simulink model "q1_adaptive_controller_simulink"  (R2019a)
settings: Solver=VariableStepAuto  StartTime=0.0  StopTime=20  RelTol=1e-3
values from neighbouring files (symbols this model uses):
  alfa_1 = L*m*g    (= 9.8)    [q1_adaptive_controller_workspce.m]
  alfa_2 = k*L^2    (= 1)    [q1_adaptive_controller_workspce.m]
  alfa_3 = c*L^2    (= 1)    [q1_adaptive_controller_workspce.m]
  gama = 5    [q1_adaptive_controller_workspce.m]
  J = 2*L^2/3*m    (= 0.666666666667)    [q1_adaptive_controller_workspce.m]
  K = 10    [q1_adaptive_controller_workspce.m]
  lamda_0 = 5    [q1_adaptive_controller_workspce.m]
  Ts = 0.001    [q1_adaptive_controller_workspce.m]
libraries: simulink x1
settings Model: Creator=ronil  LastModifiedBy=ronil

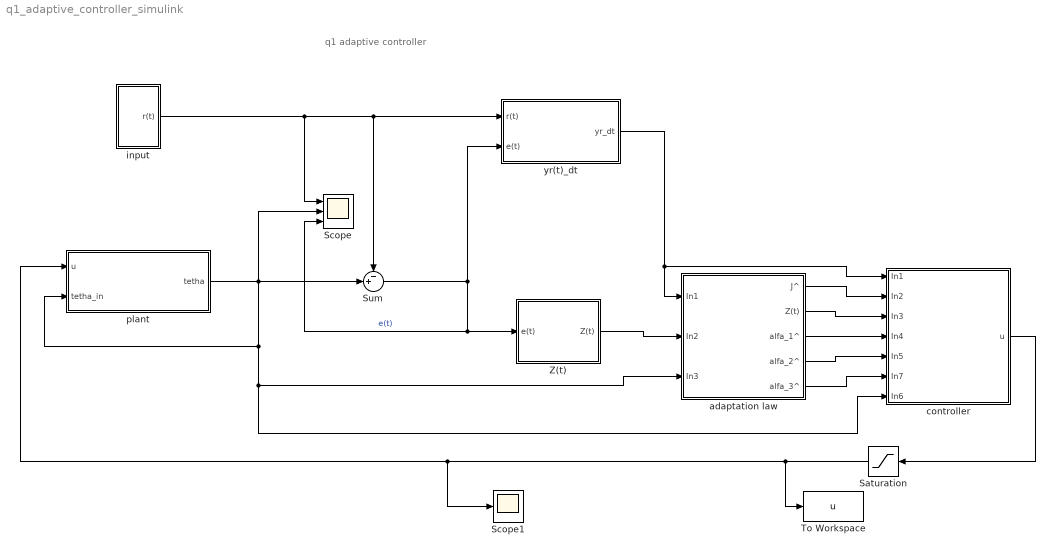
== system q1_adaptive_controller_simulink ==
  note: q1 adaptive controller
  Saturation : Saturate  UpperLimit=100000  LowerLimit=-100000  LinearizeAsGain=off  ZeroCross=off
  Scope : Scope  NumInputPorts=3
  Scope1 : Scope
  Sum : Sum  Inputs=-+|
  To Workspace : ToWorkspace  VariableName=u  SaveFormat=Timeseries  SampleTime=Ts
  Z(t) : Subsystem
  adaptation law : Subsystem
  controller : Subsystem
  input : Subsystem
  plant : Subsystem
  yr(t)_dt : Subsystem
  wires:
  plant/1(tetha) -> Scope/2, Sum/2, plant/2(tetha_in), controller/7(In6), adaptation law/3(In3)
  Sum/1 -> Z(t)/1(e(t)), Scope/3, yr(t)_dt/2(e(t))  "e(t)"
  yr(t)_dt/1(yr_dt) -> controller/1(In1), adaptation law/1(In1)
  Z(t)/1(Z(t)) -> adaptation law/2(In2)
  adaptation law/1(J^) -> controller/2(In2)
  adaptation law/2(Z(t)) -> controller/3(In3)
  adaptation law/3(alfa_1^) -> controller/4(In4)
  adaptation law/4(alfa_2^) -> controller/5(In5)
  adaptation law/5(alfa_3^) -> controller/6(In7)
  controller/1(u) -> Saturation/1
  Saturation/1 -> To Workspace/1, Scope1/1, plant/1(u)
  input/1(r(t)) -> yr(t)_dt/1(r(t)), Sum/1, Scope/1

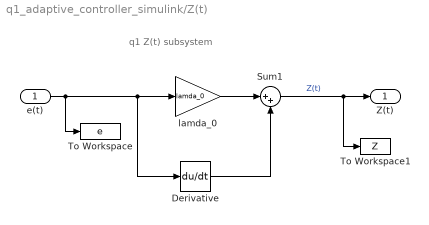
== system q1_adaptive_controller_simulink/Z(t) ==
  note: q1 Z(t) subsystem
  e(t) : Inport
  Derivative : Derivative
  Sum1 : Sum  Inputs=|++
  To Workspace : ToWorkspace  VariableName=e  SaveFormat=Timeseries  SampleTime=Ts
  To Workspace1 : ToWorkspace  VariableName=Z  SaveFormat=Timeseries  SampleTime=Ts
  lamda_0 : Gain  Gain=lamda_0
  Z(t) : Outport
  wires:
  e(t)/1 -> To Workspace/1, Derivative/1, lamda_0/1
  Derivative/1 -> Sum1/2
  Sum1/1 -> To Workspace1/1, Z(t)/1  "Z(t)"
  lamda_0/1 -> Sum1/1

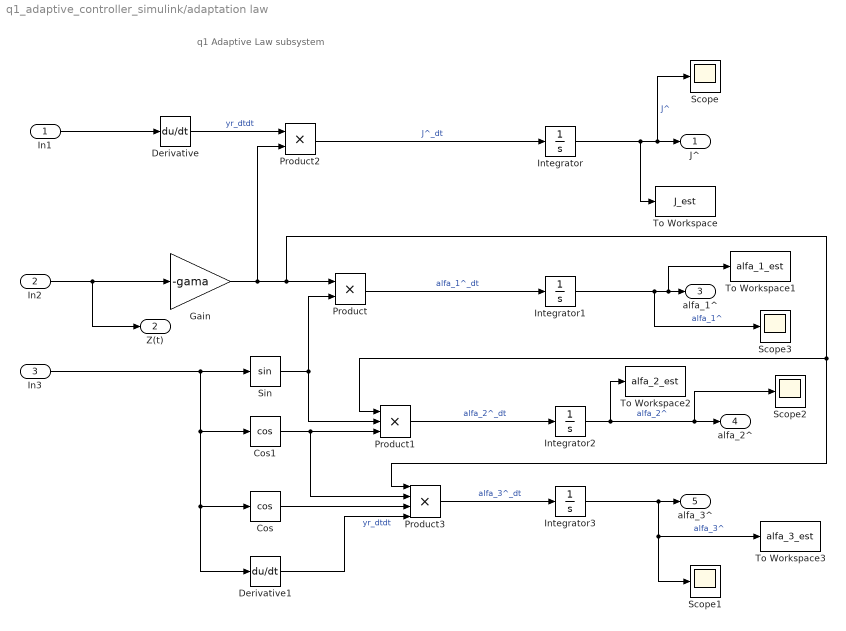
== system q1_adaptive_controller_simulink/adaptation law ==
  note: q1 Adaptive Law subsystem
  In1 : Inport
  In2 : Inport  Port=2
  In3 : Inport  Port=3
  Cos : Trigonometry  Operator=cos
  Cos1 : Trigonometry  Operator=cos
  Derivative : Derivative
  Derivative1 : Derivative
  Gain : Gain  Gain=-gama
  Integrator{,1..3} (4 alike) : Integrator
  Product : Product
  Product1 : Product  Inputs=3
  Product2 : Product
  Product3 : Product  Inputs=4
  Scope{,1..3} (4 alike) : Scope
  Sin : Trigonometry
  To Workspace : ToWorkspace  VariableName=J_est  SaveFormat=Timeseries  SampleTime=Ts
  To Workspace1 : ToWorkspace  VariableName=alfa_1_est  SaveFormat=Timeseries  SampleTime=Ts
  To Workspace2 : ToWorkspace  VariableName=alfa_2_est  SaveFormat=Timeseries  SampleTime=Ts
  To Workspace3 : ToWorkspace  VariableName=alfa_3_est  SaveFormat=Timeseries  SampleTime=Ts
  J^ : Outport
  Z(t) : Outport  Port=2
  alfa_1^ : Outport  Port=3
  alfa_2^ : Outport  Port=4
  alfa_3^ : Outport  Port=5
  wires:
  Product1/1 -> Integrator2/1  "alfa_2^_dt"
  Gain/1 -> Product2/2, Product/1, Product3/1, Product1/1
  Derivative/1 -> Product2/1  "yr_dtdt"
  Cos1/1 -> Product1/3, Product3/2
  In3/1 -> Cos/1, Derivative1/1, Cos1/1, Sin/1
  Sin/1 -> Product1/2, Product/2
  Derivative1/1 -> Product3/4  "yr_dtdt"
  Product/1 -> Integrator1/1  "alfa_1^_dt"
  Product2/1 -> Integrator/1  "J^_dt"
  Cos/1 -> Product3/3
  Product3/1 -> Integrator3/1  "alfa_3^_dt"
  In2/1 -> Z(t)/1, Gain/1
  Integrator2/1 -> To Workspace2/1, Scope2/1, alfa_2^/1  "alfa_2^"
  Integrator1/1 -> Scope3/1, To Workspace1/1, alfa_1^/1  "alfa_1^"
  Integrator3/1 -> To Workspace3/1, Scope1/1, alfa_3^/1  "alfa_3^"
  In1/1 -> Derivative/1
  Integrator/1 -> To Workspace/1, Scope/1, J^/1  "J^"

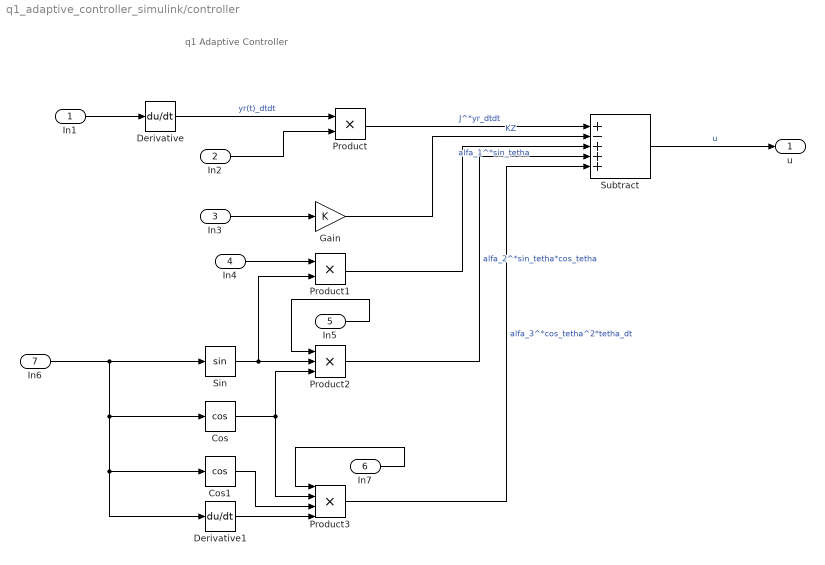
== system q1_adaptive_controller_simulink/controller ==
  note: q1 Adaptive Controller
  In1 : Inport
  In2 : Inport  Port=2
  In3 : Inport  Port=3
  In4 : Inport  Port=4
  In5 : Inport  Port=5
  In7 : Inport  Port=6
  In6 : Inport  Port=7
  Cos : Trigonometry  Operator=cos
  Cos1 : Trigonometry  Operator=cos
  Derivative : Derivative
  Derivative1 : Derivative
  Gain : Gain  Gain=K
  Product : Product
  Product1 : Product
  Product2 : Product  Inputs=3
  Product3 : Product  Inputs=4
  Sin : Trigonometry
  Subtract : Sum  Inputs=+-+++
  u : Outport
  wires:
  Product3/1 -> Subtract/5  "alfa_3^*cos_tetha^2*tetha_dt"
  Cos/1 -> Product3/2, Product2/3
  Derivative1/1 -> Product3/4
  Product2/1 -> Subtract/4  "alfa_2^*sin_tetha*cos_tetha"
  Sin/1 -> Product1/2, Product2/2
  Cos1/1 -> Product3/3
  In6/1 -> Derivative1/1, Cos1/1, Cos/1, Sin/1
  Gain/1 -> Subtract/2  "KZ"
  Derivative/1 -> Product/1  "yr(t)_dtdt"
  Product/1 -> Subtract/1  "J^*yr_dtdt"
  In2/1 -> Product/2
  Subtract/1 -> u/1  "u"
  Product1/1 -> Subtract/3  "alfa_1^*sin_tetha"
  In1/1 -> Derivative/1
  In7/1 -> Product3/1
  In3/1 -> Gain/1
  In5/1 -> Product2/1
  In4/1 -> Product1/1

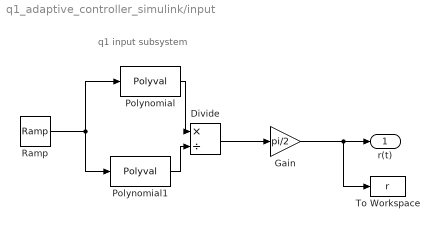
== system q1_adaptive_controller_simulink/input ==
  note: q1 input subsystem
  Divide : Product  Inputs=*/
  Gain : Gain  Gain=pi/2
  Polynomial : Polyval  Coefs=[1 0 0 0 0 0]
  Polynomial1 : Polyval  Coefs=[1 0 0 0 0 1000]
  Ramp : simulink/Sources/Ramp  slope=1  start=0  InitialOutput=0  VectorParams1D=off
  To Workspace : ToWorkspace  VariableName=r  SaveFormat=Timeseries  SampleTime=Ts
  r(t) : Outport
  wires:
  Gain/1 -> To Workspace/1, r(t)/1
  Ramp/1 -> Polynomial/1, Polynomial1/1
  Polynomial/1 -> Divide/1
  Divide/1 -> Gain/1
  Polynomial1/1 -> Divide/2

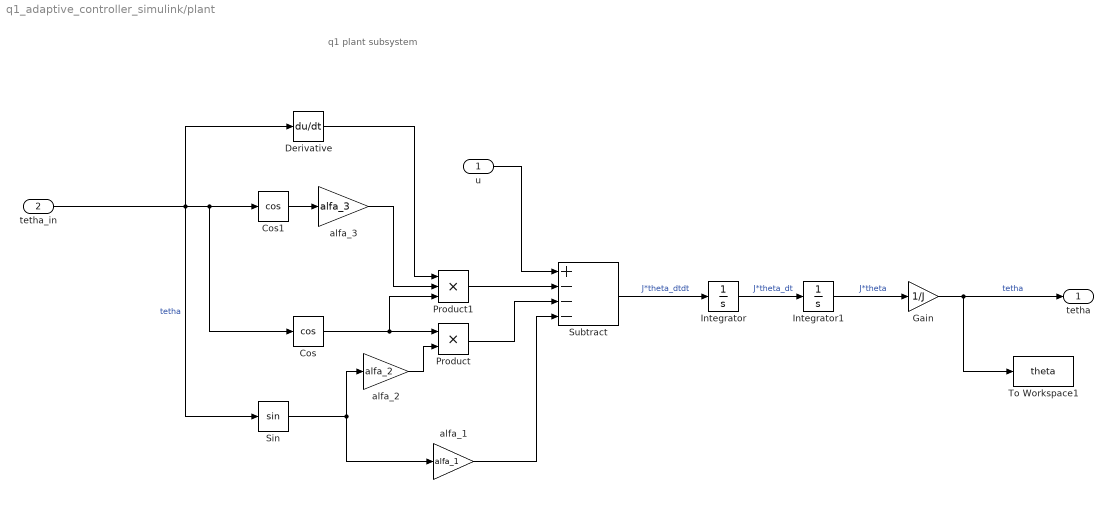
== system q1_adaptive_controller_simulink/plant ==
  note: q1 plant subsystem
  u : Inport
  tetha_in : Inport  Port=2
  Cos : Trigonometry  Operator=cos
  Cos1 : Trigonometry  Operator=cos
  Derivative : Derivative
  Gain : Gain  Gain=1/J
  Integrator : Integrator
  Integrator1 : Integrator
  Product : Product
  Product1 : Product  Inputs=3
  Sin : Trigonometry
  Subtract : Sum  Inputs=+---
  To Workspace1 : ToWorkspace  VariableName=theta  SaveFormat=Timeseries  SampleTime=Ts
  alfa_1 : Gain  Gain=alfa_1
  alfa_2 : Gain  Gain=alfa_2
  alfa_3 : Gain  Gain=alfa_3
  tetha : Outport
  wires:
  alfa_1/1 -> Subtract/4
  Integrator/1 -> Integrator1/1  "J*theta_dt"
  Cos/1 -> Product1/3, Product/1
  Gain/1 -> To Workspace1/1, tetha/1  "tetha"
  alfa_2/1 -> Product/2
  Sin/1 -> alfa_1/1, alfa_2/1
  alfa_3/1 -> Product1/2
  Cos1/1 -> alfa_3/1
  Product1/1 -> Subtract/2
  Product/1 -> Subtract/3
  Integrator1/1 -> Gain/1  "J*theta"
  Subtract/1 -> Integrator/1  "J*theta_dtdt"
  u/1 -> Subtract/1
  tetha_in/1 -> Derivative/1, Sin/1, Cos/1, Cos1/1  "tetha"
  Derivative/1 -> Product1/1

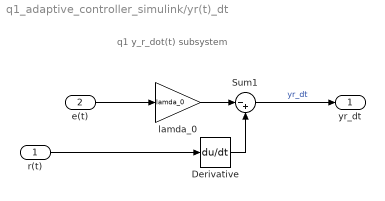
== system q1_adaptive_controller_simulink/yr(t)_dt ==
  note: q1 y_r_dot(t) subsystem
  r(t) : Inport
  e(t) : Inport  Port=2
  Derivative : Derivative
  Sum1 : Sum  Inputs=|-+
  lamda_0 : Gain  Gain=lamda_0
  yr_dt : Outport
  wires:
  lamda_0/1 -> Sum1/1
  Derivative/1 -> Sum1/2
  r(t)/1 -> Derivative/1
  e(t)/1 -> lamda_0/1
  Sum1/1 -> yr_dt/1  "yr_dt"
